simulink model "power_V2G_GA"  (R2015a)
settings: Solver=ode23tb  SolverMode=SingleTasking  StartTime=0.0  StopTime=24*60*60  RelTol=1e-4  AbsTol=1e-2
PreLoadFcn:
  | % Load Data and Parameters used by the model:
  | load power_V2G.mat
  | to=0.1;
undefined symbols (not defined in the file or in its folder): A, B, C, D1, Dd, Delta, Init, j, V2G
libraries: powerlib x54, simulink x19, simulink_extras x6, sps_avr x1, V2Glib x1, powerlib_meascontrol x1
(part 3 of 3)

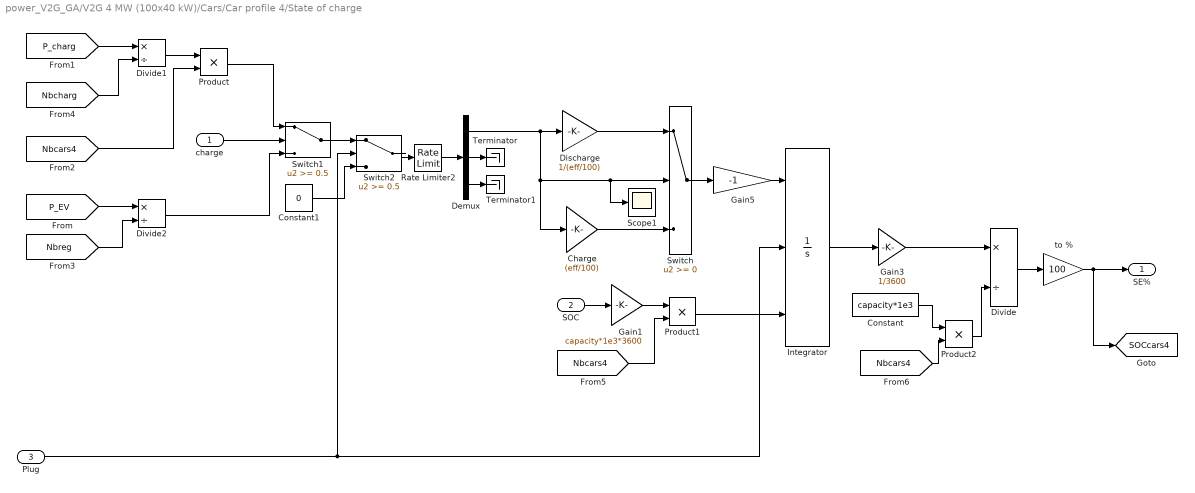
== system power_V2G_GA/V2G 4 MW (100x40 kW)/Cars/Car profile 4/State of charge ==
  charge : Inport
  SOC : Inport  Port=2
  Plug : Inport  Port=3
  Charge : Gain  Gain=(eff/100)
  Constant : Constant  Value=capacity*1e3
  Constant1 : Constant  Value=0
  Demux : Demux  Outputs=3
  Discharge : Gain  Gain=1/(eff/100)
  Divide : Product  Inputs=*/
  Divide1 : Product  Inputs=*/
  Divide2 : Product  Inputs=*/
  Gain1 : Gain  Gain=capacity*1e3*3600
  Gain3 : Gain  Gain=1/3600
  Gain5 : Gain  Gain=-1
  Integrator : Integrator  ExternalReset=either  InitialConditionSource=external  InitialCondition=Init*850e3*3600
  Product : Product
  Product1 : Product
  Product2 : Product
  Rate Limiter2 : RateLimiter  RisingSlewLimit=1e4  FallingSlewLimit=-1e4  SampleTimeMode=inherited
  Scope1 : Scope
      settings: YMin=-466  YMax=-453  SaveName=ScopeData19
  Switch : Switch  ZeroCross=off
  Switch1 : Switch  Threshold=0.5  ZeroCross=off
  Switch2 : Switch  Threshold=0.5  ZeroCross=off
  Terminator : Terminator
  Terminator1 : Terminator
  to % : Gain  Gain=100
  SE% : Outport
  tag scope: SOCcars4=global
  wires:
  Discharge/1 -> Switch/1
  Charge/1 -> Switch/3
  Switch/1 -> Gain5/1
  Gain5/1 -> Integrator/1
  Integrator/1 -> Gain3/1
  Divide/1 -> to %/1
  Gain3/1 -> Divide/1
  to %/1 -> [SOCcars4], SE%/1
  Demux/2 -> Terminator/1
  Demux/3 -> Terminator1/1
  Plug/1 -> Integrator/2, Switch2/2
  SOC/1 -> Gain1/1
  charge/1 -> Switch1/2
  Demux/1 -> Charge/1, Scope1/1, Switch/2, Discharge/1
  [P_charg] -> Divide1/1
  [Nbreg] -> Divide2/2
  [P_EV] -> Divide2/1
  [Nbcharg] -> Divide1/2
  Divide1/1 -> Product/1
  [Nbcars4] -> Product/2
  Product/1 -> Switch1/1
  Divide2/1 -> Switch1/3
  Switch1/1 -> Switch2/1
  Constant1/1 -> Switch2/3
  Switch2/1 -> Rate Limiter2/1
  [Nbcars4] -> Product1/2
  Gain1/1 -> Product1/1
  Product1/1 -> Integrator/3
  Product2/1 -> Divide/2
  [Nbcars4] -> Product2/2
  Constant/1 -> Product2/1
  Rate Limiter2/1 -> Demux/1

== system power_V2G_GA/V2G 4 MW (100x40 kW)/Cars/Car profile 5/Charger control ==
  SE% : Inport
  "Plug " : Inport  Port=2
  Compare To Constant : simulink/Logic and Bit Operations/Compare To Constant  relop=<=  const=85  OutDataTypeStr=boolean
  Compare To Constant1 : simulink/Logic and Bit Operations/Compare To Constant  relop=>=  const=95  OutDataTypeStr=boolean
  Logical Operator : Logic  AllPortsSameDT=off  OutDataTypeStr=boolean
  Logical Operator1 : Logic  Operator=NOT  AllPortsSameDT=off  OutDataTypeStr=boolean
  Logical Operator2 : Logic  AllPortsSameDT=off  OutDataTypeStr=boolean
  S-R Flip-Flop : simulink_extras/Flip Flops/S-R Flip-Flop  initial_condition=0
  Terminator : Terminator
  "Charge mode " : Outport
  "Regulation mode " : Outport  Port=2
  wires:
  S-R Flip-Flop/2 -> Terminator/1
  Logical Operator1/1 -> Logical Operator2/1
  Logical Operator2/1 -> "Regulation mode "/1
  Logical Operator/1 -> "Charge mode "/1
  S-R Flip-Flop/1 -> Logical Operator/1, Logical Operator1/1
  "Plug "/1 -> Logical Operator/2, Logical Operator2/2
  Compare To Constant1/1 -> S-R Flip-Flop/2
  Compare To Constant/1 -> S-R Flip-Flop/1
  SE%/1 -> Compare To Constant/1, Compare To Constant1/1

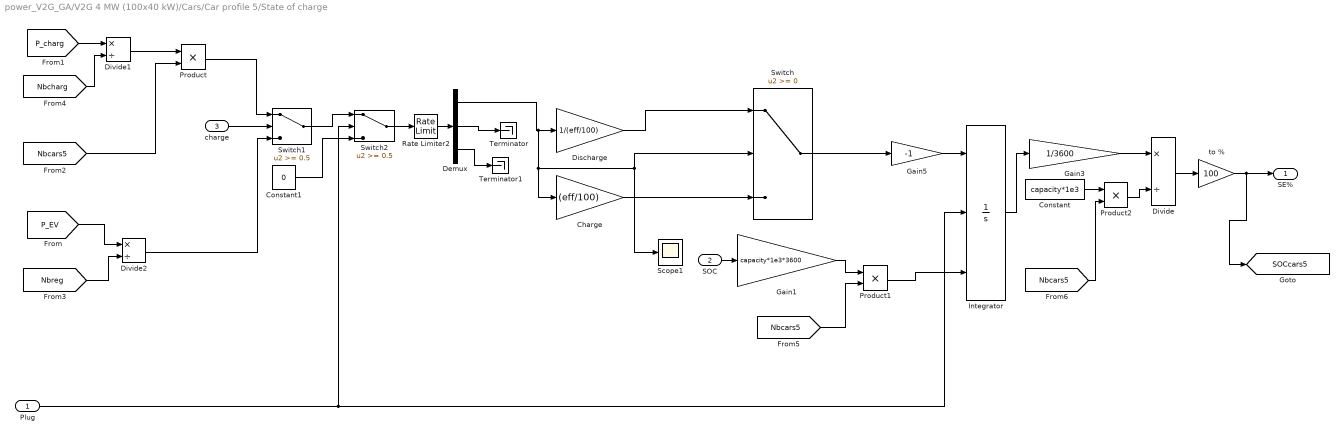
== system power_V2G_GA/V2G 4 MW (100x40 kW)/Cars/Car profile 5/State of charge ==
  Plug : Inport
  SOC : Inport  Port=2
  charge : Inport  Port=3
  Charge : Gain  Gain=(eff/100)
  Constant : Constant  Value=capacity*1e3
  Constant1 : Constant  Value=0
  Demux : Demux  Outputs=3
  Discharge : Gain  Gain=1/(eff/100)
  Divide : Product  Inputs=*/
  Divide1 : Product  Inputs=*/
  Divide2 : Product  Inputs=*/
  Gain1 : Gain  Gain=capacity*1e3*3600
  Gain3 : Gain  Gain=1/3600
  Gain5 : Gain  Gain=-1
  Integrator : Integrator  ExternalReset=either  InitialConditionSource=external  InitialCondition=Init*850e3*3600
  Product : Product
  Product1 : Product
  Product2 : Product
  Rate Limiter2 : RateLimiter  RisingSlewLimit=1e4  FallingSlewLimit=-1e4  SampleTimeMode=inherited
  Scope1 : Scope
      settings: YMin=-210000  YMax=10000  SaveName=ScopeData19
  Switch : Switch  ZeroCross=off
  Switch1 : Switch  Threshold=0.5  ZeroCross=off
  Switch2 : Switch  Threshold=0.5  ZeroCross=off
  Terminator : Terminator
  Terminator1 : Terminator
  to % : Gain  Gain=100
  SE% : Outport
  tag scope: SOCcars5=global
  wires:
  Rate Limiter2/1 -> Demux/1
  Product2/1 -> Divide/2
  Constant/1 -> Product2/1
  [Nbcars5] -> Product2/2
  Product1/1 -> Integrator/3
  [Nbcars5] -> Product1/2
  Gain1/1 -> Product1/1
  Switch2/1 -> Rate Limiter2/1
  Constant1/1 -> Switch2/3
  Switch1/1 -> Switch2/1
  Divide2/1 -> Switch1/3
  Product/1 -> Switch1/1
  [Nbcars5] -> Product/2
  Divide1/1 -> Product/1
  [Nbcharg] -> Divide1/2
  [P_EV] -> Divide2/1
  [Nbreg] -> Divide2/2
  [P_charg] -> Divide1/1
  Demux/1 -> Discharge/1, Charge/1, Switch/2, Scope1/1
  charge/1 -> Switch1/2
  SOC/1 -> Gain1/1
  Plug/1 -> Switch2/2, Integrator/2
  Demux/3 -> Terminator1/1
  Demux/2 -> Terminator/1
  to %/1 -> SE%/1, [SOCcars5]
  Gain3/1 -> Divide/1
  Divide/1 -> to %/1
  Integrator/1 -> Gain3/1
  Gain5/1 -> Integrator/1
  Switch/1 -> Gain5/1
  Charge/1 -> Switch/3
  Discharge/1 -> Switch/1

== system power_V2G_GA/V2G 4 MW (100x40 kW)/Charge power generation/Break Alg. Loop 2/imag ==
  In1 : Inport
  State Space : StateSpace  A=A  B=B  C=C  D=Dd  X0=X0
  Out1 : Outport  InitialOutput=0
  wires:
  State Space/1 -> Out1/1
  In1/1 -> State Space/1

== system power_V2G_GA/V2G 4 MW (100x40 kW)/Charge power generation/Break Alg. Loop 2/real ==
  In1 : Inport
  State Space : StateSpace  A=A  B=B  C=C  D=Dd  X0=X0
  Out1 : Outport  InitialOutput=0
  wires:
  State Space/1 -> Out1/1
  In1/1 -> State Space/1

== system power_V2G_GA/V2G 4 MW (100x40 kW)/Grid regulation/Grid regulation power  generation/Avoid division by zero ==
  I : Inport
  Complex to Magnitude-Angle : ComplexToMagnitudeAngle
  Magnitude-Angle to Complex : MagnitudeAngleToComplex
  Saturation1 : Saturate  UpperLimit=inf  LowerLimit=1e-6
  O : Outport
  wires:
  I/1 -> Complex to Magnitude-Angle/1
  Saturation1/1 -> Magnitude-Angle to Complex/1
  Complex to Magnitude-Angle/1 -> Saturation1/1
  Magnitude-Angle to Complex/1 -> O/1
  Complex to Magnitude-Angle/2 -> Magnitude-Angle to Complex/2

== system power_V2G_GA/V2G 4 MW (100x40 kW)/Grid regulation/Grid regulation power  generation/Break Alg. Loop 1 ==
  In : Inport
  Complex to Real-Imag : ComplexToRealImag
  Real-Imag to Complex : RealImagToComplex
  imag : Subsystem  mask(Transfer Function with Initial Outputs){N=[1], D=[to  1], Y0=0, U0=0}
      mask prompts: N "Numerator:"; D "Denominator:"; Y0 "Initial output:"; U0 "Initial input:"
      mask help: Vector expressions for numerator, and denominator. Coefficients are in descending powers of s.
      mask init:
      | [A,B,C,Dd]=tf2ss(N,D);if (isempty(Y0));[m,n]=size(A);X0=zeros(1,m); end; if (isempty(U0));[m,p]=size(B);U0=zeros(1,p);end;X0=getxo(A,B,C,Dd,U0,Y0,0);
      mask Help: Specify the initial output for the transfer function.  An optimization routine attempts to determine the appropriate initial states so that the specified initial output is achieved.  For more details, see the m-file getxo.m
      mask Display: dpoly(N,D,'s')
  real : Subsystem  mask(Transfer Function with Initial Outputs){N=[1], D=[to 1], Y0=0, U0=0}
      mask prompts: N "Numerator:"; D "Denominator:"; Y0 "Initial output:"; U0 "Initial input:"
      mask help: Vector expressions for numerator, and denominator. Coefficients are in descending powers of s.
      mask init:
      | [A,B,C,Dd]=tf2ss(N,D);if (isempty(Y0));[m,n]=size(A);X0=zeros(1,m); end; if (isempty(U0));[m,p]=size(B);U0=zeros(1,p);end;X0=getxo(A,B,C,Dd,U0,Y0,0);
      mask Help: Specify the initial output for the transfer function.  An optimization routine attempts to determine the appropriate initial states so that the specified initial output is achieved.  For more details, see the m-file getxo.m
      mask Display: dpoly(N,D,'s')
  Out : Outport
  wires:
  Complex to Real-Imag/1 -> real/1(In1)
  Complex to Real-Imag/2 -> imag/1(In1)
  In/1 -> Complex to Real-Imag/1
  Real-Imag to Complex/1 -> Out/1
  real/1(Out1) -> Real-Imag to Complex/1
  imag/1(Out1) -> Real-Imag to Complex/2

== system power_V2G_GA/Wind Farm 4.5 MW/Wind Farm/Break Alg. Loop 1/imag ==
  In1 : Inport
  State Space : StateSpace  A=A  B=B  C=C  D=Dd  X0=X0
  Out1 : Outport  InitialOutput=0
  wires:
  State Space/1 -> Out1/1
  In1/1 -> State Space/1

== system power_V2G_GA/Wind Farm 4.5 MW/Wind Farm/Break Alg. Loop 1/real ==
  In1 : Inport
  State Space : StateSpace  A=A  B=B  C=C  D=Dd  X0=X0
  Out1 : Outport  InitialOutput=0
  wires:
  State Space/1 -> Out1/1
  In1/1 -> State Space/1

== system power_V2G_GA/V2G 4 MW (100x40 kW)/Grid regulation/Grid regulation power  generation/Break Alg. Loop 1/imag ==
  In1 : Inport
  State Space : StateSpace  A=A  B=B  C=C  D=Dd  X0=X0
  Out1 : Outport  InitialOutput=0
  wires:
  State Space/1 -> Out1/1
  In1/1 -> State Space/1

== system power_V2G_GA/V2G 4 MW (100x40 kW)/Grid regulation/Grid regulation power  generation/Break Alg. Loop 1/real ==
  In1 : Inport
  State Space : StateSpace  A=A  B=B  C=C  D=Dd  X0=X0
  Out1 : Outport  InitialOutput=0
  wires:
  State Space/1 -> Out1/1
  In1/1 -> State Space/1
